simulink model "pendulum_model"  (R2024a)
settings: Solver=ode1  StartTime=0.0  StopTime=10.0  FixedStep=0.001  RelTol=1e-3
undefined symbols (not defined in the file or in its folder): a, b, d, K, lambda, phi
settings Model: Creator=Lenovo  LastModifiedBy=Lenovo
settings DataIOCC: ReturnWorkspaceOutputs=off

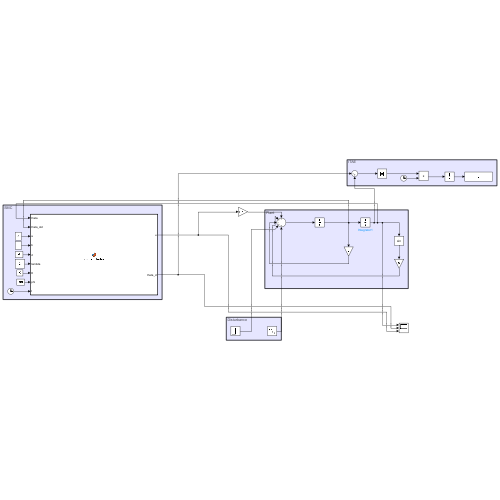
[thumbnail: Simulink's stored preview of the top-level diagram]
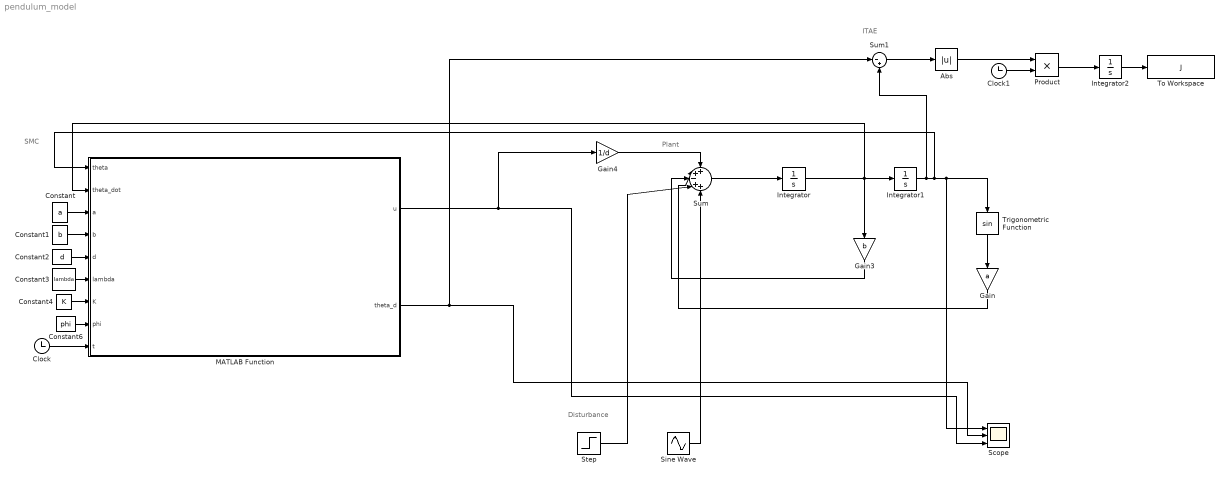
== system pendulum_model ==
  note: Disturbance
  note: ITAE
  note: SMC
  note: Plant
  Abs : Abs  SaturateOnIntegerOverflow=off
  Clock : Clock
  Clock1 : Clock
  Constant : Constant  Value=a
  Constant1 : Constant  Value=b
  Constant2 : Constant  Value=d
  Constant3 : Constant  Value=lambda
  Constant4 : Constant  Value=K
  Constant6 : Constant  Value=phi
  Gain : Gain  Gain=a
  Gain3 : Gain  Gain=b
  Gain4 : Gain  Gain=1/d
  Integrator : Integrator
  Integrator1 : Integrator  InitialCondition=2
  Integrator2 : Integrator
  MATLAB Function : MATLAB Function  TreatAsAtomicUnit=on
  Product : Product
  Scope : Scope  NumInputPorts=3
  Sine Wave : Sin  Amplitude=17  Frequency=3  SampleTime=0
  Step : Step  Time=4  After=15  SampleTime=0
  Sum : Sum  Inputs=++-++
  Sum1 : Sum  Inputs=|-+
  To Workspace : ToWorkspace  VariableName=J  SampleTime=-1
  Trigonometric Function : Trigonometry
  wires:
  Gain/1 -> Sum/2
  Gain3/1 -> Sum/3
  Sum/1 -> Integrator/1
  Trigonometric Function/1 -> Gain/1
  Gain4/1 -> Sum/1
  MATLAB Function/1(u) -> Scope/3, Gain4/1
  Integrator/1 -> MATLAB Function/2(theta_dot), Gain3/1, Integrator1/1
  Constant6/1 -> MATLAB Function/8(phi)
  Constant1/1 -> MATLAB Function/4(b)
  Constant3/1 -> MATLAB Function/6(lambda)
  Clock/1 -> MATLAB Function/9(t)
  Constant4/1 -> MATLAB Function/7(K)
  Constant2/1 -> MATLAB Function/5(d)
  Constant/1 -> MATLAB Function/3(a)
  Step/1 -> Sum/4
  Sine Wave/1 -> Sum/5
  Integrator2/1 -> To Workspace/1
  Sum1/1 -> Abs/1
  Integrator1/1 -> Trigonometric Function/1, Scope/1, MATLAB Function/1(theta), Sum1/2
  MATLAB Function/2(theta_d) -> Sum1/1, Scope/2
  Product/1 -> Integrator2/1
  Clock1/1 -> Product/2
  Abs/1 -> Product/1

== matlab function pendulum_model/MATLAB Function ==
  data: theta input; u output; theta_dot input; a input; b input; d input; lambda input; K input; phi input; t input; theta_d output
function [u, theta_d] = smc_controller(theta, theta_dot, a, b, d, lambda, K, phi, t)
theta_d = 0;
theta_d_dot = 0;
theta_d_dot_dot = 0;
e = theta - theta_d;
e_dot = theta_dot - theta_d_dot;
s = e_dot + lambda*e;
u_eq = (1/d)*(theta_d_dot_dot - a*sin(theta) + b*theta_dot - lambda*e_dot);
u_sw=(-K/d)*(s/(abs(s)+phi));
u = u_eq + u_sw;
